simulink model "dc_motor_control_test"  (R2021a)
settings: Solver=ode45  StartTime=0.0  StopTime=40  RelTol=1e-3  EnableMultiTasking=on
values from neighbouring files (symbols this model uses):
  adingain = [adingain 1 1 1 1 1]    [hwinit.m]
  adinoffs = [adinoffs 0 0 0 0 0]    [hwinit.m]
  daoutgain = 1*[-6]    [hwinit.m]
  daoutoffs = [0.00]    [hwinit.m]
  h = 0.01    [Linearization_4state.m]    (also in hwinit.m = 0.001; rotpentest.m = fugiboard('Open', 'pendulum1'))
  K = model.Km    [Linearization_4state.m]    (also in Model_derivation.m = K_trans + K_rot; Model_derivation_4_states.m = K_trans + K_rot; dc_motor_control.m = dlqr(dt_sys_zoh.A, dt_sys_zoh.B, Q_lqr, R_lqr); identification_dc_motor.m = -0.05)
  K_ff = 1/dcgain_sys    [dc_motor_control.m]    (also in rotating_pendulum_3states.m; rotating_pendulum_4states.m)
  R_kf = 1 * diag([1, 10, 1, 10])    [dc_motor_control.m]    (also in rotating_pendulum_3states.m = 10 * diag([1, 1, 10]); rotating_pendulum_4states.m = diag([7.5740e-06, 0.1526, 1.4489e-05, 0.2930]))
undefined symbols (not defined in the file or in its folder): Discrete, Time
libraries: ctrlSharedLib x1
settings Model: Creator=rbabuska  LastModifiedBy=danny
settings SolverCC: AlgebraicLoopSolver=TrustRegion
settings DataIOCC: LimitDataPoints=on  SaveFormat=Array  ReturnWorkspaceOutputs=off  SignalLoggingName=sigsOut
settings OptimizationCC: BooleanDataType=off  ExpressionDepthLimit=2147483647  InitFltsAndDblsToZero=on  LifeSpan=inf
settings DebuggingCC: SaveWithParameterizedLinksMsg=none  SignalResolutionControl=TryResolveAllWithWarning  MultiTaskDSMMsg=warning  MultiTaskCondExecSysMsg=none  AllowSymbolicDim=off  StateNameClashWarn=warning  SFUnexpectedBacktrackingDiag=warning  SFNoUnconditionalDefaultTransitionDiag=warning  SFExecutionAtInitializationDiag=none  SFMachineParentedDataDiag=warning  ArithmeticOperatorsInVariantConditions=warning
settings HardwareCC: ProdBitPerPointer=32  ProdBitPerSizeT=32  ProdBitPerPtrDiffT=32  ProdLargestAtomicFloat=None  ProdIntDivRoundTo=Undefined  ProdEndianess=Unspecified  ProdWordSize=32  ProdHWDeviceType=32-bit Generic  TargetUnknown=on
settings ModelReferenceCC: PropagateSignalLabelsOutOfModel=off
settings SFSimCC: SimUseLocalCustomCode=off  CustomCodeUndefinedFunction=UseInterfaceOnly
settings RTWCC: RTWUseLocalCustomCode=off
settings CodeAppCC: StateflowObjectComments=on
settings GRTTargetCC: TargetFcnLib=ansi_tfl_tmw.mat  TargetLangStandard=C89/C90 (ANSI)  CombineOutputUpdateFcns=off  GRTInterface=on
settings ConfigComp: CovMetricSettings=dw  CovSaveCumulativeToWorkspaceVar=on  CovSaveSingleToWorkspaceVar=on  CovExternalEMLEnable=off

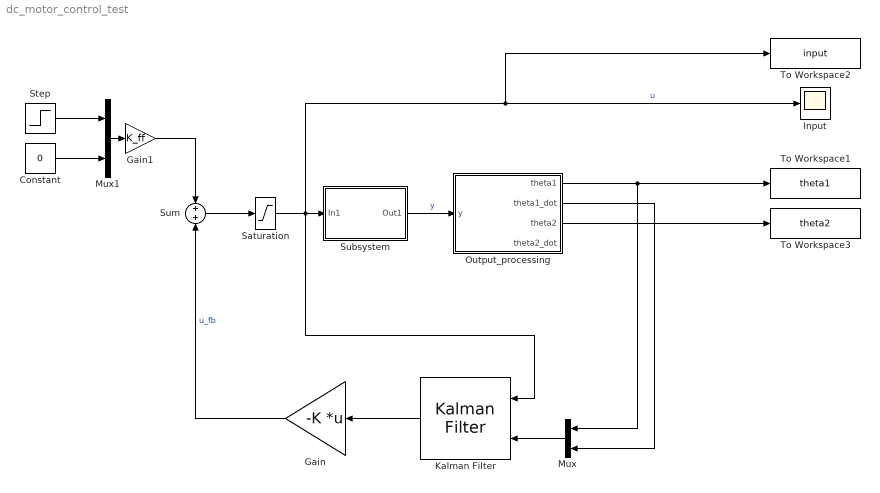
== system dc_motor_control_test ==
  Constant : Constant  Value=0
  Gain : Gain  Gain=-K  Multiplication=Matrix(K*u)
  Gain1 : Gain  Gain=K_ff
  Input : Scope
  Kalman Filter : ctrlSharedLib/Kalman Filter  TimeDomain=Discrete-Time  UseCurrentEstimator=on  ModelSource=LTI State-Space Variable  ModelSourceVariable=dc_motor_ss  A=0.95  B=1  C=1  D=0  NumberOfStates=1  NumberOfInputs=1  NumberOfOutputs=1  InitialEstimateSource=Dialog  X0=0  P0=10  UseK=off  UseGH=off  NumberOfProcessNoiseInputs=1  G=1  TimeInvariantG=on  H=0  TimeInvariantH=on  Q=Q_kf  TimeInvariantQ=on  R=R_kf  TimeInvariantR=on  N=0  TimeInvariantN=on  AddInputPort=on  AddEnablePort=off  OutputEstimatedY=off  OutputP=off  Ts=-1
  Mux : Mux  Inputs=2
  Mux1 : Mux  Inputs=2
  Output_processing : Subsystem
  Saturation : Saturate  UpperLimit=1  LowerLimit=-1
  Step : Step  Time=2  SampleTime=0
  Subsystem : Subsystem
      mask Display: disp('Rotational\nPendulum')
  Sum : Sum  Inputs=+|+
  To Workspace1 : ToWorkspace  VariableName=theta1  SaveFormat=Timeseries  SampleTime=-1
  To Workspace2 : ToWorkspace  VariableName=input  SaveFormat=Timeseries  SampleTime=-1
  To Workspace3 : ToWorkspace  VariableName=theta2  SaveFormat=Timeseries  SampleTime=-1
  wires:
  Saturation/1 -> Subsystem/1(In1), To Workspace2/1, Input/1, Kalman Filter/1  "u"
  Mux/1 -> Kalman Filter/2
  Kalman Filter/1 -> Gain/1
  Subsystem/1(Out1) -> Output_processing/1(y)  "y"
  Output_processing/1(theta1) -> Mux/1, To Workspace1/1
  Output_processing/3(theta2) -> To Workspace3/1
  Output_processing/2(theta1_dot) -> Mux/2
  Step/1 -> Mux1/1
  Constant/1 -> Mux1/2
  Mux1/1 -> Gain1/1
  Sum/1 -> Saturation/1
  Gain/1 -> Sum/2  "u_fb"
  Gain1/1 -> Sum/1

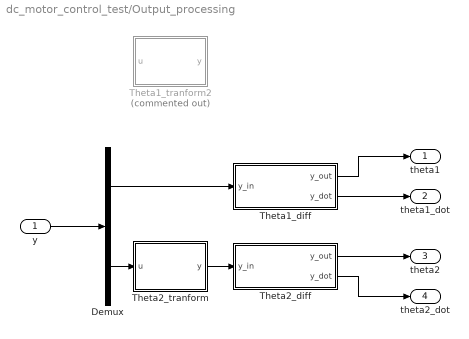
== system dc_motor_control_test/Output_processing ==
  y : Inport
  Demux : Demux  Outputs=2
  Theta1_diff : Subsystem
  Theta1_tranform2 : MATLAB Function  Commented=on  TreatAsAtomicUnit=on
  Theta2_diff : Subsystem
  Theta2_tranform : MATLAB Function  TreatAsAtomicUnit=on
  theta1 : Outport
  theta1_dot : Outport  Port=2
  theta2 : Outport  Port=3
  theta2_dot : Outport  Port=4
  wires:
  y/1 -> Demux/1
  Theta2_diff/1(y_out) -> theta2/1
  Theta1_diff/2(y_dot) -> theta1_dot/1
  Demux/1 -> Theta1_diff/1(y_in)
  Theta2_tranform/1(y) -> Theta2_diff/1(y_in)
  Demux/2 -> Theta2_tranform/1(u)
  Theta2_diff/2(y_dot) -> theta2_dot/1
  Theta1_diff/1(y_out) -> theta1/1

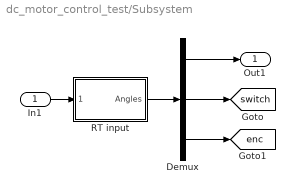
== system dc_motor_control_test/Subsystem ==
  In1 : Inport
  Demux : Demux  Outputs=[2 4 1]
  RT input : Subsystem  mask{Ts=h, channels=[6 7]}
      mask prompts: Ts "Sample time [s]:"; channels "Channels to read (e.g., [6 7])"
      mask init:
      | hwinit;
      | 
      | % initialize FPGA
      | fugihandle = fugiboard('Open', 'Pendulum1');
      | fugihandle.WatchdogTimeout = 0.5;
      | fugiboard('SetParams', fugihandle);
      | fugiboard('Write', fugihandle, 0, 0, 0, 0);  % dummy write to sync interface board
      | fugiboard('Write', fugihandle, 5, 1, 0, 0);  % reset position, activate relay
      | data = fugiboard('Read', fugihandle);        % get version info from FPGA
      | % model = bitshift(data(1), -5); 
      | % version = bitand(data(1), 31);
      | % disp(sprintf('FPGA setup %d, version %d', model, version)); % for the B&P it should say 1 1, or else there is a problem
      | fugiboard('Write', fugihandle, 0, 1, 0, 0);  % end reset
      | pause(0.1);                         % give relay some time to respond
      mask Display: disp('Rotational\nPendulum')
  Out1 : Outport
  tag scope: enc=global, switch=global
  wires:
  RT input/1(Angles) -> Demux/1
  Demux/1 -> Out1/1
  Demux/2 -> [switch]
  Demux/3 -> [enc]
  In1/1 -> RT input/1(Motors)

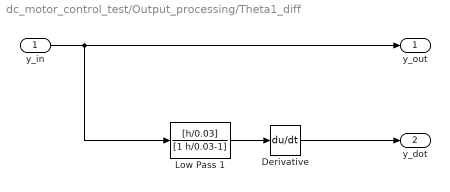
== system dc_motor_control_test/Output_processing/Theta1_diff ==
  y_in : Inport
  Derivative : Derivative
  Low Pass 1 : DiscreteTransferFcn  Numerator=[h/0.03]  Denominator=[1 h/0.03-1]
  y_out : Outport
  y_dot : Outport  Port=2
  wires:
  y_in/1 -> Low Pass 1/1, y_out/1
  Derivative/1 -> y_dot/1
  Low Pass 1/1 -> Derivative/1

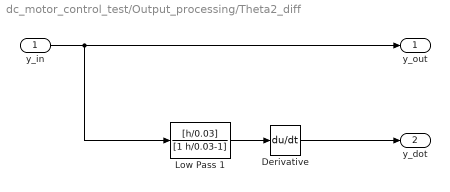
== system dc_motor_control_test/Output_processing/Theta2_diff ==
  y_in : Inport
  Derivative : Derivative
  Low Pass 1 : DiscreteTransferFcn  Numerator=[h/0.03]  Denominator=[1 h/0.03-1]
  y_out : Outport
  y_dot : Outport  Port=2
  wires:
  Low Pass 1/1 -> Derivative/1
  Derivative/1 -> y_dot/1
  y_in/1 -> y_out/1, Low Pass 1/1

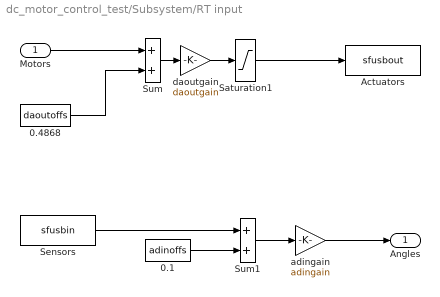
== system dc_motor_control_test/Subsystem/RT input ==
  Motors : Inport
  0.1 : Constant  Value=adinoffs
  0.4868 : Constant  Value=daoutoffs
  Actuators : S-Function  FunctionName=sfusbout  Parameters=Ts, fugihandle  SFunctionDeploymentMode=off  EnableBusSupport=off
  Saturation1 : Saturate  UpperLimit=10  LowerLimit=-10
  Sensors : S-Function  FunctionName=sfusbin  Parameters=Ts, fugihandle, channels  SFunctionDeploymentMode=off  EnableBusSupport=off
  Sum : Sum  InputSameDT=on  SaturateOnIntegerOverflow=on  OutDataTypeStr=Inherit: Same as first input
  Sum1 : Sum  InputSameDT=on  SaturateOnIntegerOverflow=on  OutDataTypeStr=Inherit: Same as first input
  adingain : Gain  Gain=adingain  SaturateOnIntegerOverflow=on  OutDataTypeStr=Inherit: Same as input  ParamDataTypeStr=Inherit: Same as input
  daoutgain : Gain  Gain=daoutgain  SaturateOnIntegerOverflow=on  OutDataTypeStr=Inherit: Same as input  ParamDataTypeStr=Inherit: Same as input
  Angles : Outport
  wires:
  Sum/1 -> daoutgain/1
  0.4868/1 -> Sum/2
  Motors/1 -> Sum/1
  Sum1/1 -> adingain/1
  0.1/1 -> Sum1/2
  adingain/1 -> Angles/1
  Saturation1/1 -> Actuators/1
  daoutgain/1 -> Saturation1/1
  Sensors/1 -> Sum1/1

== matlab function dc_motor_control_test/Output_processing/Theta2_tranform ==
  data: u input; y output
function y = fcn(u)
if (u<0)
    u = u+2*pi;
end
u=u-pi;
y = u;

== matlab function dc_motor_control_test/Output_processing/Theta1_tranform2 ==
  data: u input; y output
function y = fcn2(u)
if (u<0)
    u = u+2*pi;
end
y = u-pi;
